simulink model "Control_Trayectoria"  (R2020b)
settings: Solver=FixedStepAuto  StartTime=0.0  StopTime=T_final  FixedStep=0.02  RelTol=1e-3  EnableMultiTasking=on
values from neighbouring files (symbols this model uses):
  theta_init = pi/4    (= 0.785398163397)    [Prueba_trayectoria.m]
  x_init = -e*cos(theta_init)    [Prueba_trayectoria.m]
  y_init = -e*sin(theta_init)    [Prueba_trayectoria.m]
libraries: simulink x1
settings Model: Creator=rausifer  LastModifiedBy=alexa
settings DataIOCC: LimitDataPoints=on  SaveFormat=Array  ReturnWorkspaceOutputs=off
settings OptimizationCC: ExpressionDepthLimit=2147483647  LifeSpan=inf
settings DebuggingCC: UnderspecifiedInitializationDetection=Classic  MergeDetectMultiDrivingBlocksExec=none  SolverPrmCheckMsg=warning  FcnCallInpInsideContextMsg=warning  StateNameClashWarn=warning  SFUnexpectedBacktrackingDiag=warning  SFNoUnconditionalDefaultTransitionDiag=warning  SFExecutionAtInitializationDiag=none  ArithmeticOperatorsInVariantConditions=warning
settings HardwareCC: ProdBitPerPointer=32  ProdBitPerSizeT=32  ProdBitPerPtrDiffT=32  ProdLargestAtomicFloat=None  ProdIntDivRoundTo=Undefined  ProdEndianess=Unspecified  ProdWordSize=32  ProdHWDeviceType=32-bit Generic
settings ModelReferenceCC: PropagateSignalLabelsOutOfModel=off
settings SFSimCC: SimUseLocalCustomCode=off  CustomCodeUndefinedFunction=UseInterfaceOnly
settings RTWCC: RTWUseLocalCustomCode=off
settings CodeAppCC: StateflowObjectComments=on
settings GRTTargetCC: TargetLangStandard=C89/C90 (ANSI)  CombineOutputUpdateFcns=off  GRTInterface=on
settings ConfigComp: CovMetricSettings=dw  CovSaveCumulativeToWorkspaceVar=on  CovSaveSingleToWorkspaceVar=on  CovExternalEMLEnable=off  CovSFcnEnable=off

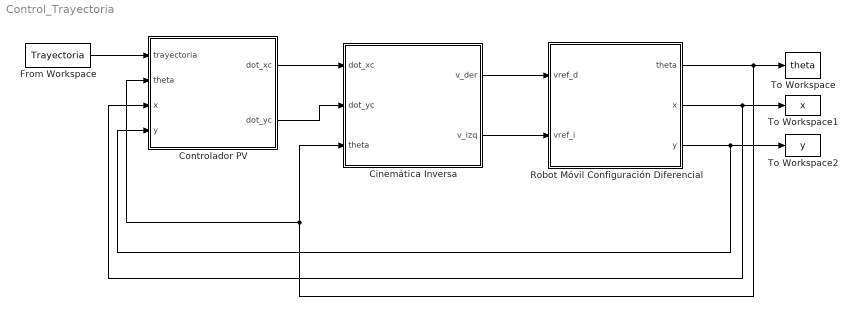
== system Control_Trayectoria ==
  Cinemática Inversa : MATLAB Function  TreatAsAtomicUnit=on
  Controlador PV : MATLAB Function  TreatAsAtomicUnit=on
  From Workspace : FromWorkspace  VariableName=Trayectoria  SampleTime=0.02  OutputAfterFinalValue=Holding final value
  Robot Móvil Configuración Diferencial : Subsystem
  To Workspace : ToWorkspace  VariableName=theta  SampleTime=-1
  To Workspace1 : ToWorkspace  VariableName=x  SampleTime=-1
  To Workspace2 : ToWorkspace  VariableName=y  SampleTime=-1
  wires:
  Robot Móvil Configuración Diferencial/2(x) -> Controlador PV/3(x), To Workspace1/1
  Cinemática Inversa/1(v_der) -> Robot Móvil Configuración Diferencial/1(vref_d)
  Cinemática Inversa/2(v_izq) -> Robot Móvil Configuración Diferencial/2(vref_i)
  Robot Móvil Configuración Diferencial/1(theta) -> To Workspace/1, Cinemática Inversa/3(theta), Controlador PV/2(theta)
  From Workspace/1 -> Controlador PV/1(trayectoria)
  Robot Móvil Configuración Diferencial/3(y) -> Controlador PV/4(y), To Workspace2/1
  Controlador PV/2(dot_yc) -> Cinemática Inversa/2(dot_yc)
  Controlador PV/1(dot_xc) -> Cinemática Inversa/1(dot_xc)

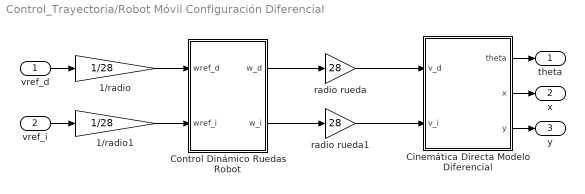
== system Control_Trayectoria/Robot Móvil Configuración Diferencial ==
  vref_d : Inport
  vref_i : Inport  Port=2
  1/radio : Gain  Gain=1/28
  1/radio1 : Gain  Gain=1/28
  Cinemática Directa Modelo Diferencial : Subsystem
  Control Dinámico Ruedas Robot : Subsystem
  radio rueda : Gain  Gain=28
  radio rueda1 : Gain  Gain=28
  theta : Outport  VectorParamsAs1DForOutWhenUnconnected=off
  x : Outport  Port=2  VectorParamsAs1DForOutWhenUnconnected=off
  y : Outport  Port=3  VectorParamsAs1DForOutWhenUnconnected=off
  wires:
  1/radio/1 -> Control Dinámico Ruedas Robot/1(wref_d)
  1/radio1/1 -> Control Dinámico Ruedas Robot/2(wref_i)
  Control Dinámico Ruedas Robot/1(w_d) -> radio rueda/1
  Control Dinámico Ruedas Robot/2(w_i) -> radio rueda1/1
  radio rueda/1 -> Cinemática Directa Modelo Diferencial/1(v_d)
  radio rueda1/1 -> Cinemática Directa Modelo Diferencial/2(v_i)
  Cinemática Directa Modelo Diferencial/1(theta) -> theta/1
  vref_d/1 -> 1/radio/1
  Cinemática Directa Modelo Diferencial/2(x) -> x/1
  vref_i/1 -> 1/radio1/1
  Cinemática Directa Modelo Diferencial/3(y) -> y/1

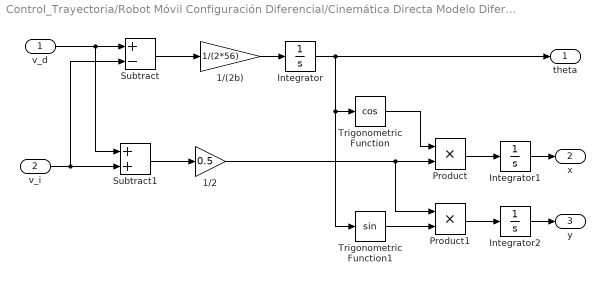
== system Control_Trayectoria/Robot Móvil Configuración Diferencial/Cinemática Directa Modelo Diferencial ==
  v_d : Inport
  v_i : Inport  Port=2
  1/(2b) : Gain  Gain=1/(2*56)
  1/2 : Gain  Gain=0.5
  Integrator : Integrator  InitialCondition=theta_init
  Integrator1 : Integrator  InitialCondition=x_init
  Integrator2 : Integrator  InitialCondition=y_init
  Product : Product  RndMeth=Zero
  Product1 : Product  RndMeth=Zero
  Subtract : Sum  Inputs=+-
  Subtract1 : Sum
  Trigonometric Function : Trigonometry  Operator=cos
  Trigonometric Function1 : Trigonometry
  theta : Outport  VectorParamsAs1DForOutWhenUnconnected=off
  x : Outport  Port=2  VectorParamsAs1DForOutWhenUnconnected=off
  y : Outport  Port=3  VectorParamsAs1DForOutWhenUnconnected=off
  wires:
  v_d/1 -> Subtract1/1, Subtract/1
  v_i/1 -> Subtract/2, Subtract1/2
  Subtract/1 -> 1/(2b)/1
  Subtract1/1 -> 1/2/1
  1/(2b)/1 -> Integrator/1
  Integrator/1 -> Trigonometric Function/1, Trigonometric Function1/1, theta/1
  Trigonometric Function/1 -> Product/1
  1/2/1 -> Product/2, Product1/1
  Product/1 -> Integrator1/1
  Product1/1 -> Integrator2/1
  Trigonometric Function1/1 -> Product1/2
  Integrator1/1 -> x/1
  Integrator2/1 -> y/1

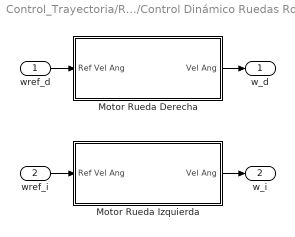
== system Control_Trayectoria/Robot Móvil Configuración Diferencial/Control Dinámico Ruedas Robot ==
  wref_d : Inport
  wref_i : Inport  Port=2
  Motor Rueda Derecha : Subsystem  mask(Controlador y modelo de motor rueda Lego EV3){k=0.146, tau=0.0634, ruido=off, Kp=3.4754, Ti=0.0463, Td=.005}
      mask prompts: k "Valor ganancia motor"; tau "Valor tiempo motor"; Kp "Valor Kp"; Ti "Valor Ti"; Td "Valor Td"
      mask help: Este bloque incluye un bloque de funcion de controlador tipo PID discreto que hay que implementar (en ecuaciones en diferencias). Ademas incluye el modelo del motor de una rueda de Lego EV3, al que se le pueden cambiar los valores para personalizarlo.
      mask DialogControl ParameterGroupVar Prompt: Parámetros
  Motor Rueda Izquierda : Subsystem  mask(Controlador y modelo de motor rueda Lego EV3){k=0.146, tau=0.0634, ruido=off, Kp=3.4754, Ti=0.0463, Td=.005}
      mask prompts: k "Valor ganancia motor"; tau "Valor tiempo motor"; Kp "Valor Kp"; Ti "Valor Ti"; Td "Valor Td"
      mask help: Este bloque incluye un bloque de funcion de controlador tipo PID discreto que hay que implementar (en ecuaciones en diferencias). Ademas incluye el modelo del motor de una rueda de Lego EV3, al que se le pueden cambiar los valores para personalizarlo.
      mask DialogControl ParameterGroupVar Prompt: Parámetros
  w_d : Outport  VectorParamsAs1DForOutWhenUnconnected=off
  w_i : Outport  Port=2  VectorParamsAs1DForOutWhenUnconnected=off
  wires:
  wref_d/1 -> Motor Rueda Derecha/1(Ref Vel Ang)
  Motor Rueda Derecha/1(Vel Ang) -> w_d/1
  wref_i/1 -> Motor Rueda Izquierda/1(Ref Vel Ang)
  Motor Rueda Izquierda/1(Vel Ang) -> w_i/1

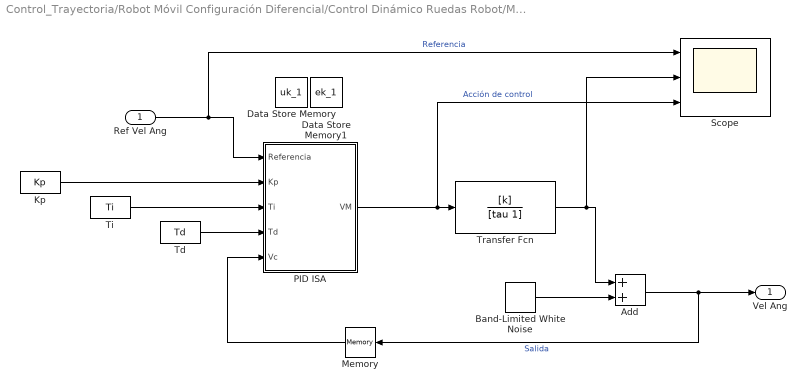
== system Control_Trayectoria/Robot Móvil Configuración Diferencial/Control Dinámico Ruedas Robot/Motor Rueda Derecha ==
  Ref Vel Ang : Inport
  Add : Sum
  Band-Limited White Noise : simulink/Sources/Band-Limited White Noise  Cov=[0.002]*ruido  Ts=0.02  seed=[23341]
  Data Store Memory : DataStoreMemory  DataStoreName=uk_1  ReadBeforeWriteMsg=warning  WriteAfterWriteMsg=warning  WriteAfterReadMsg=warning  ShowAdditionalParam=off  OutDataTypeStr=double
  Data Store Memory1 : DataStoreMemory  DataStoreName=ek_1  ReadBeforeWriteMsg=warning  WriteAfterWriteMsg=warning  WriteAfterReadMsg=warning  ShowAdditionalParam=off  OutDataTypeStr=double
  Kp : Constant  Value=Kp
  Memory : Memory  InheritSampleTime=on
  PID ISA : MATLAB Function  TreatAsAtomicUnit=on  SystemSampleTime=0.02
      settings: MinAlgLoopOccurrences=on
  Scope : Scope  NumInputPorts=3
  Td : Constant  Value=Td
  Ti : Constant  Value=Ti
  Transfer Fcn : TransferFcn  Numerator=[k]  Denominator=[tau 1]
  Vel Ang : Outport  VectorParamsAs1DForOutWhenUnconnected=off
  wires:
  Add/1 -> Vel Ang/1, Memory/1  "Salida"
  Ti/1 -> PID ISA/3(Ti)
  PID ISA/1(VM) -> Scope/3, Transfer Fcn/1  "Acción de control"
  Memory/1 -> PID ISA/5(Vc)
  Td/1 -> PID ISA/4(Td)
  Kp/1 -> PID ISA/2(Kp)
  Ref Vel Ang/1 -> Scope/1, PID ISA/1(Referencia)  "Referencia"
  Band-Limited White Noise/1 -> Add/2
  Transfer Fcn/1 -> Scope/2, Add/1

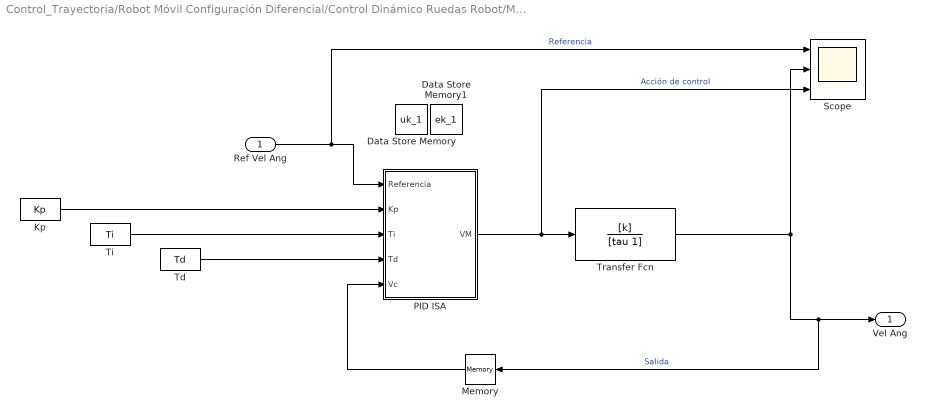
== system Control_Trayectoria/Robot Móvil Configuración Diferencial/Control Dinámico Ruedas Robot/Motor Rueda Izquierda ==
  Ref Vel Ang : Inport
  Data Store Memory : DataStoreMemory  DataStoreName=uk_1  ReadBeforeWriteMsg=warning  WriteAfterWriteMsg=warning  WriteAfterReadMsg=warning  ShowAdditionalParam=off  OutDataTypeStr=double
  Data Store Memory1 : DataStoreMemory  DataStoreName=ek_1  ReadBeforeWriteMsg=warning  WriteAfterWriteMsg=warning  WriteAfterReadMsg=warning  ShowAdditionalParam=off  OutDataTypeStr=double
  Kp : Constant  Value=Kp
  Memory : Memory  InheritSampleTime=on
  PID ISA : MATLAB Function  TreatAsAtomicUnit=on  SystemSampleTime=0.02
      settings: MinAlgLoopOccurrences=on
  Scope : Scope  NumInputPorts=3
  Td : Constant  Value=Td
  Ti : Constant  Value=Ti
  Transfer Fcn : TransferFcn  Numerator=[k]  Denominator=[tau 1]
  Vel Ang : Outport  VectorParamsAs1DForOutWhenUnconnected=off
  wires:
  Ref Vel Ang/1 -> Scope/1, PID ISA/1(Referencia)  "Referencia"
  Kp/1 -> PID ISA/2(Kp)
  Td/1 -> PID ISA/4(Td)
  Memory/1 -> PID ISA/5(Vc)
  PID ISA/1(VM) -> Scope/3, Transfer Fcn/1  "Acción de control"
  Ti/1 -> PID ISA/3(Ti)
  Transfer Fcn/1 -> Scope/2, Memory/1, Vel Ang/1  "Salida"

== matlab function Control_Trayectoria/Robot Móvil Configuración Diferencial/Control Dinámico Ruedas Robot/Motor Rueda Derecha/PID ISA ==
  data: Referencia input; Kp input; Ti input; Td input; VM output; Vc input; uk_1 data_store_memory; ek_1 data_store_memory
function VM = PID(Referencia,Kp,Ti,Td,Vc)
Ts = 0.02;
global uk_1 ek_1;

% Calcular el Error
ek = Referencia - Vc;
% Calcular la Acción de control
up = Kp*ek;
ui = uk_1 + (Kp/Ti)*ek*Ts;
ud = Kp*Td*((ek - ek_1)/Ts);
uk =  up + ui + ud;

%Saturar la Acción de Control (-10,+10)
if (uk >= (100))
    uk = 100;
    ui = uk_1;
end     
if (uk <= (-100))
    uk = -100;
    ui = uk_1;
end

% Sumamos Punto Funcionamiento a la Accion de Control
VM = uk;

% Actualizar variables
uk_1 = ui;
ek_1 = ek;

== matlab function Control_Trayectoria/Robot Móvil Configuración Diferencial/Control Dinámico Ruedas Robot/Motor Rueda Izquierda/PID ISA ==
  data: Referencia input; Kp input; Ti input; Td input; VM output; Vc input; uk_1 data_store_memory; ek_1 data_store_memory
function VM = PID(Referencia,Kp,Ti,Td,Vc)
Ts = 0.02;
global uk_1 ek_1;

% Calcular el Error
ek = Referencia - Vc;
% Calcular la Acción de control
up = Kp*ek;
ui = uk_1 + (Kp/Ti)*ek*Ts;
ud = Kp*Td*((ek - ek_1)/Ts);
uk =  up + ui + ud;

%Saturar la Acción de Control (-10,+10)
if (uk >= (100))
    uk = 100;
    ui = uk_1;
end     
if (uk <= (-100))
    uk = -100;
    ui = uk_1;
end

% Sumamos Punto Funcionamiento a la Accion de Control
VM = uk;

% Actualizar variables
uk_1 = ui;
ek_1 = ek;

== matlab function Control_Trayectoria/Controlador PV ==
  data: trayectoria input; dot_xc output; theta input; dot_yc output; x input; y input
%Controlador Proporcional Velocidad
function [dot_xc, dot_yc] = Controlador_pv(trayectoria,theta, x, y)

    %Ley de Control cinemático Proporcional con pre-alimentación de velocidad
    %del punto de centrado en función de la configuración del robot (x,y,theta)

    %Declaración de Variables 
    Kx = 4.5; %Ganancia con respecto al error en x 
    Ky = 4.5; %Ganancia con respecto al error en y
    e = 100;%Distancia entre el punto descentralizado y el punto medio de las ruedas
    ref = trayectoria(1:2); %Trayectoria de x,y
    dot_ref = trayectoria(3:4); %Derivadas de x,y de la trayectoría
    m_ganancia = [Kx 0; 0 Ky]; %Matriz constante de ganancia
  
    %Matriz de derivadas de x,y de la trayectoría
    m_dot_ref = [dot_ref(1);dot_ref(2)];

    %Matriz del error del punto de centrado
    e1 = ref(1) - (x + e*cos(theta)); % Primer elemento de la matriz
    e2 = ref(2) - (y + e*sin(theta)); % Segundo elemento de la matriz
    m_error_punto_centrado = [e1;e2];

    % Se múltiplican para obtener los valores de XC, YC
    m_dot_xyc = m_dot_ref + m_ganancia * m_error_punto_centrado;

    %Derivadas de la trayectoría con respecto a la velocidad para x,y 
    dot_xc = m_dot_xyc(1);
    dot_yc = m_dot_xyc(2);
    
end

== matlab function Control_Trayectoria/Cinemática Inversa ==
  data: dot_xc input; v_der output; dot_yc input; theta input; v_izq output
function [v_der, v_izq] = Cinematica_Inversa(dot_xc,dot_yc,theta)

    %Declaración de Variables
    e = 100; % Distancia entre el punto descentralizado y el punto medio de las ruedas
    b = 56; % Distancia entre las ruedas
    
    %Cinemática Inversa del Punto Descentralizado
    m_vels_punto_descentralizado = [dot_xc; dot_yc];
    m_cinematica_inv = [(cos(theta)+(b/e)*sin(theta))  (sin(theta)-(b/e)*cos(theta));...
          (cos(theta)-(b/e)*sin(theta)) (sin(theta)+(b/e)*cos(theta)) ];
    m_velocidades = 1/2 * m_cinematica_inv * m_vels_punto_descentralizado;

    %Velocidades de referencia del motor
    v_izq = m_velocidades(1);
    v_der = m_velocidades(2);

end
